simulink model "model"  (R2023b)
settings: Solver=FixedStepAuto  StartTime=0.0  StopTime=10.0  FixedStep=0.0005  RelTol=1e-3
values from neighbouring files (symbols this model uses):
  dm = 0.00001    (= 1e-05)    [params.m]
  Jm = 0.0003    [params.m]
settings Model: Creator=matte  LastModifiedBy=86180
settings SolverCC: AlgebraicLoopSolver=TrustRegion
settings DebuggingCC: ArithmeticOperatorsInVariantConditions=warning
settings SFSimCC: LegacyBehaviorForPersistentVarInContinuousTime=on  CustomCodeUndefinedFunction=UseInterfaceOnly

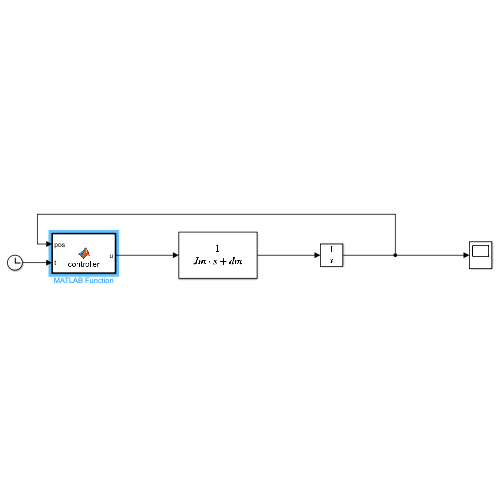
[thumbnail: Simulink's stored preview of the top-level diagram]
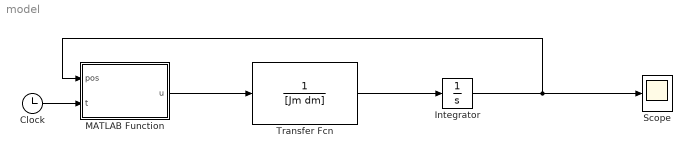
== system model ==
  Clock : Clock
  Integrator : Integrator
  MATLAB Function : MATLAB Function  TreatAsAtomicUnit=on
  Scope : Scope
  Transfer Fcn : TransferFcn  Denominator=[Jm dm]
  wires:
  Integrator/1 -> MATLAB Function/1(pos), Scope/1
  Transfer Fcn/1 -> Integrator/1
  Clock/1 -> MATLAB Function/2(t)
  MATLAB Function/1(u) -> Transfer Fcn/1

== matlab function model/MATLAB Function ==
  data: pos input; u output; t input
function u = controller(pos, t)

persistent last_t;
persistent last_pos;
persistent ie;


% One time variable initialization --------
if isempty(last_t)
    last_t = 0;
end
% ----------------------------------------

if isempty(ie)
    ie = 0;
end

dt = t - last_t;

% Dirty fix to avoid division by zero --------
if dt == 0
    dt = 1e-4;
end

% --------------------------------------------
% implement your controller here
% -------------------------------------------- 
ref = 1;


vel = (pos-last_pos)/dt
vel_e = ref - vel;
Pv=
Iv=
ie=ie+vel_e*dt;
vel_controller= Pv*vel_e + Iv*ie;
u = 0.02 * e;
last_t = t;
last_pos=pos;
